simulink model "SimulatorLQRmodel"  (R2024b)
settings: Solver=VariableStepAuto  StartTime=0.0  StopTime=10.0  RelTol=1e-3
values from neighbouring files (symbols this model uses):
  input_noise_power = 1    [CalculateBestInputs.m]    (also in SimulatorLQG.m = 10; SimulatorLQR.m = 10)
  K = lqr(A, B, Qr, Rr)    [CalculateBestInputs.m]    (also in IP_MACRO.m; LAB2_Analyze_system.m; SimulatorLQG.m; SimulatorLQR.m)
  output_noise_power = 100    [CalculateBestInputs.m]    (also in SimulatorLQG.m = 10; SimulatorLQR.m = 10)
  use_input_noise = 0    [CalculateBestInputs.m]    (also in SimulatorLQG.m = 1; SimulatorLQR.m)
  use_output_noise = 10    [CalculateBestInputs.m]    (also in SimulatorLQG.m = 1; SimulatorLQR.m = 0)
  x0 = [pi/2 0 0.1 0 0].'    [CalculateBestInputs.m]    (also in SimulatorLQG.m; SimulatorLQR.m = [0.3 0 0.1 0 0].')
undefined symbols (not defined in the file or in its folder): A, B, C, D
libraries: simulink x2
settings Model: Creator=ricar  LastModifiedBy=ricar

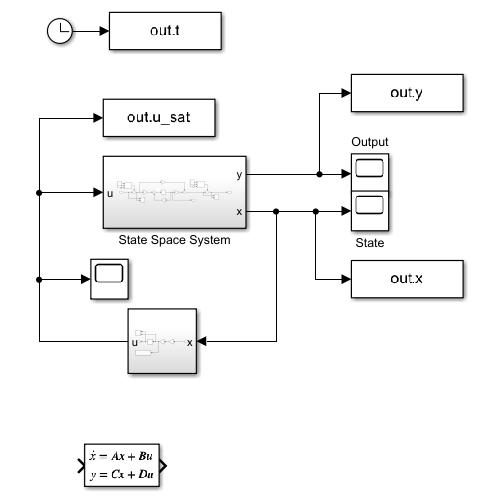
[thumbnail: Simulink's stored preview of the top-level diagram]
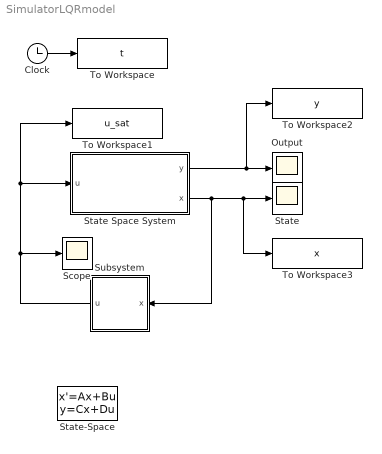
== system SimulatorLQRmodel ==
  Clock : Clock
  Output : Scope
  Scope : Scope
  State : Scope
  State Space System : Subsystem
  State-Space : StateSpace  A=A  B=B  C=C  D=D  InitialCondition=0
  Subsystem : Subsystem
  To Workspace : ToWorkspace  VariableName=t  SampleTime=-1
  To Workspace1 : ToWorkspace  VariableName=u_sat  SampleTime=-1
  To Workspace2 : ToWorkspace  VariableName=y  SampleTime=-1
  To Workspace3 : ToWorkspace  VariableName=x  SampleTime=-1
  wires:
  State Space System/1(y) -> To Workspace2/1, Output/1
  State Space System/2(x) -> Subsystem/1(x), To Workspace3/1, State/1
  Clock/1 -> To Workspace/1
  Subsystem/1(u) -> Scope/1, State Space System/1(u), To Workspace1/1

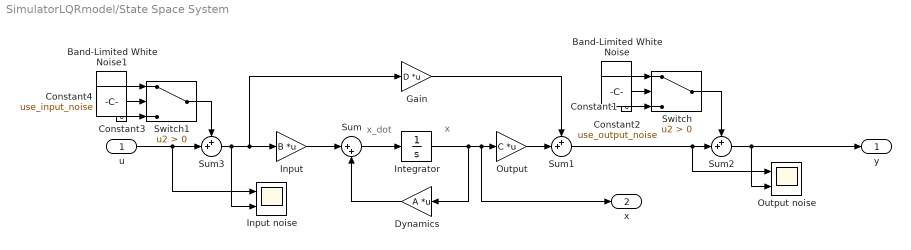
== system SimulatorLQRmodel/State Space System ==
  note: x_dot
  note: x
  u : Inport
  Band-Limited White Noise : simulink/Sources/Band-Limited White Noise  Cov=[0.000001*output_noise_power 0.000001*output_noise_power]  Ts=0.005  seed=[23341 2]
  Band-Limited White Noise1 : simulink/Sources/Band-Limited White Noise  Cov=[0.00001*input_noise_power]  Ts=0.01  seed=[145]
  Constant1 : Constant  Value=0
  Constant2 : Constant  Value=use_output_noise
  Constant3 : Constant  Value=0
  Constant4 : Constant  Value=use_input_noise
  Dynamics : Gain  Gain=A  Multiplication=Matrix(K*u)
  Gain : Gain  Gain=D  Multiplication=Matrix(K*u)
  Input : Gain  Gain=B  Multiplication=Matrix(K*u)
  Input noise : Scope  NumInputPorts=2
  Integrator : Integrator  InitialCondition=x0
  Output : Gain  Gain=C  Multiplication=Matrix(K*u)
  Output noise : Scope  NumInputPorts=2
  Sum : Sum  Inputs=|++
  Sum1 : Sum  Inputs=++|
  Sum2 : Sum  Inputs=++|
  Sum3 : Sum  Inputs=++|
  Switch : Switch  Criteria=u2 > Threshold  SaturateOnIntegerOverflow=off  InputSameDT=off
  Switch1 : Switch  Criteria=u2 > Threshold  SaturateOnIntegerOverflow=off  InputSameDT=off
  y : Outport
  x : Outport  Port=2
  wires:
  Sum/1 -> Integrator/1
  Integrator/1 -> Dynamics/1, x/1, Output/1
  Input/1 -> Sum/1
  Dynamics/1 -> Sum/2
  Output/1 -> Sum1/2
  Gain/1 -> Sum1/1
  Sum1/1 -> Output noise/1, Sum2/2
  Sum2/1 -> Output noise/2, y/1
  Switch/1 -> Sum2/1
  Constant2/1 -> Switch/2
  Band-Limited White Noise/1 -> Switch/1
  Constant1/1 -> Switch/3
  Constant4/1 -> Switch1/2
  Switch1/1 -> Sum3/1
  Constant3/1 -> Switch1/3
  Band-Limited White Noise1/1 -> Switch1/1
  Sum3/1 -> Input noise/2, Gain/1, Input/1
  u/1 -> Input noise/1, Sum3/2

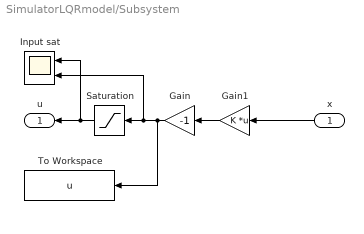
== system SimulatorLQRmodel/Subsystem ==
  x : Inport
  Gain : Gain  Gain=-1
  Gain1 : Gain  Gain=K  Multiplication=Matrix(K*u)
  Input sat : Scope  NumInputPorts=2
  Saturation : Saturate  UpperLimit=5  LowerLimit=-5
  To Workspace : ToWorkspace  VariableName=u  SaveFormat=Timeseries  SampleTime=-1
  u : Outport
  wires:
  Gain1/1 -> Gain/1
  x/1 -> Gain1/1
  Saturation/1 -> Input sat/1, u/1
  Gain/1 -> To Workspace/1, Input sat/2, Saturation/1
